simulink model "Simscape_simulink"  (R2024a)
settings: Solver=VariableStepAuto  StartTime=0.0  StopTime=10.0  MaxStep=0.001  RelTol=1e-3
libraries: fl_lib x15, nesl_utility x6, sdl_lib x1
settings Model: Creator=buttrakd  LastModifiedBy=buttrakd

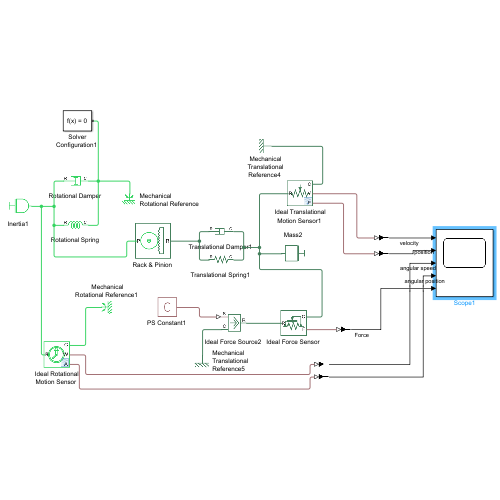
[thumbnail: Simulink's stored preview of the top-level diagram]
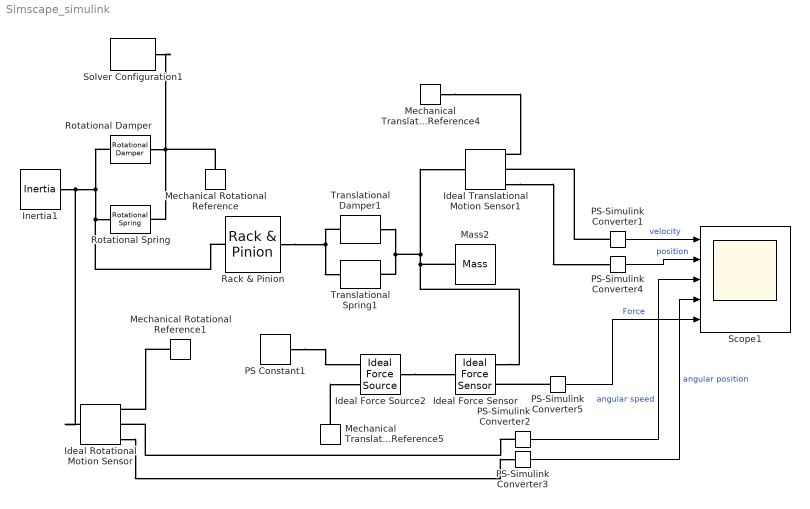
== system Simscape_simulink ==
  "Ideal Force Sensor " : fl_lib/Mechanical/Mechanical Sensors/Ideal Force Sensor
  "Ideal Force Source2 " : fl_lib/Mechanical/Mechanical Sources/Ideal Force Source
  "Ideal Rotational Motion Sensor " : fl_lib/Mechanical/Mechanical Sensors/Ideal Rotational Motion Sensor  reference=foundation.enum.MeasurementReference.difference  acceleration_port=false  velocity_port=true  position_port=true  wrap_angle=false  offset=0 rad
      settings: SimscapeInstrumentationLogging=on
  "Ideal Translational Motion Sensor1 " : fl_lib/Mechanical/Mechanical Sensors/Ideal Translational Motion Sensor  reference=foundation.enum.MeasurementReference.difference  acceleration_port=false  velocity_port=true  position_port=true  offset=0 m
      settings: SimscapeInstrumentationLogging=on
  "Inertia1 " : fl_lib/Mechanical/Rotational Elements/Inertia  inertia=1 kg*m^2  num_ports=foundation.enum.numPorts2.one  w_specify=off  w_priority=High  w=0 rad/s  w_nominal_specify=off  w_nominal_value=1  w_nominal_unit=rad/s  t_specify=off  t_priority=None  t=0 N*m  t_nominal_specify=off  t_nominal_value=1  t_nominal_unit=N*m
  "Mass2 " : fl_lib/Mechanical/Translational Elements/Mass  mass=0.5 kg  num_ports=foundation.enum.numPorts2.one  v_specify=off  v_priority=High  v=0 m/s  v_nominal_specify=off  v_nominal_value=1  v_nominal_unit=m/s  f_specify=off  f_priority=None  f=0 N  f_nominal_specify=off  f_nominal_value=1  f_nominal_unit=N
  "Mechanical Rotational Reference " : fl_lib/Mechanical/Rotational Elements/Mechanical Rotational Reference
  "Mechanical Rotational Reference1 " : fl_lib/Mechanical/Rotational Elements/Mechanical Rotational Reference
  "Mechanical Translational Reference4 " : fl_lib/Mechanical/Translational Elements/Mechanical Translational Reference
  "Mechanical Translational Reference5 " : fl_lib/Mechanical/Translational Elements/Mechanical Translational Reference
  "PS Constant1 " : fl_lib/Physical Signals/Sources/PS Constant  constant=1 N
  PS-Simulink Converter{1..5} (5 alike) : nesl_utility/PS-Simulink Converter  PhysicalDomain=network_engine_domain  SubClassName=ps_output  LeftPortType=input  RightPortType=output  PseudoPeriodic=off  Frequencies=[]  VectorFormat=inherit  Unit=inherit  AffineConversion=off
  "Rack & Pinion " : sdl_lib/Gears/Rotational- Translational/Rack & Pinion  param=sdl.enum.rackPinionParameters.radius  radius=0.4 m  n_teeth=20  x_tooth=5 mm  rack_direction_sign=sdl.enum.pinionDirection.positive  friction_model=sdl.enum.gear_friction.none  efficiency=0.8  temperature_TLU=[280, 300, 320] K  efficiency_TLU=[.95, .9, .85]  pwr_thr=0.001 W  mu_visc_P=0 N*m*s/rad  mu_visc_R=0 N*s/m  thermal_mass=50 J/K  temperature_specify=off  temperature_priority=High  temperature=300 K  temperature_nominal_specify=off  temperature_nominal_value=1  temperature_nominal_unit=K
      settings: InternalSimscapePortConfiguration="{\"Bottom\":[],\"Left\":[{\"id\":\"P\",\"label\":\"P\",\"type\":\"foundation.mechanical.rotational.rotational\"}],\"Right\":[{\"id\":\"R\",\"label\":\"R\",\"type\":\"foundation.mechanical.translational.translational\"}],\"Top\":[]}"
  "Rotational Damper " : fl_lib/Mechanical/Rotational Elements/Rotational Damper  D=0.25 N*m*s/rad  w_specify=off  w_priority=None  w=0 rad/s  w_nominal_specify=off  w_nominal_value=1  w_nominal_unit=rad/s  t_specify=off  t_priority=None  t=0 N*m  t_nominal_specify=off  t_nominal_value=1  t_nominal_unit=N*m
  "Rotational Spring " : fl_lib/Mechanical/Rotational Elements/Rotational Spring  spr_rate=0.5 N*m/rad  w_specify=off  w_priority=None  w=0 rad/s  w_nominal_specify=off  w_nominal_value=1  w_nominal_unit=rad/s  t_specify=off  t_priority=None  t=0 N*m  t_nominal_specify=off  t_nominal_value=1  t_nominal_unit=N*m  phi_specify=off  phi_priority=High  phi=0 rad  phi_nominal_specify=off  phi_nominal_value=1  phi_nominal_unit=rad
  Scope1 : Scope  NumInputPorts=5
  "Solver Configuration1 " : nesl_utility/Solver Configuration  PhysicalDomain=network_engine_domain  SubClassName=solver  LeftPortType=input  RightPortType=generic  Tones=[]  Harmonics=[]  SimulateNoise=off  Profile=off  UseLocalSampling=off  EnableSwitchedLinearOptims=on  FrequencyDomain=off  UseCCode=off  RelTol=0.001  AbsTol=0.001  MinStep=1e-09  ToWorkspace=off  RevertToSquareIcSolve=off  NumHomotopyIterations=100  PhasorMode=off  PhasorModeNumHarmonics=1  ConsistencySolver=NEWTON_XTOL_AFTER_FTOL  IndexReductionMethod=DerivativeReplacement  DoDC=off  ResidualTolerance=1e-09  ConsistencyTolSource=GLOBAL  ConsistencyAbsTol=0.001  ConsistencyRelTol=0.001  ConsistencyTolFactor=0.001  UseLocalSolver=off  LocalSolverChoice=NE_BACKWARD_EULER_ADVANCER  ResolveIndetEquations=on  FunctionEvalNumThread=1  LocalSolverSampleTime=0.001  DoFixedCost=off  MaxNonlinIter=3  MaxModeIter=2  ComputeImpulses=off  ImpulseIterations=2  LinearAlgebra=auto  LinearAlgebraNumThread=0  EquationFormulation=NE_TIME_EF  DelaysMemoryBudget=1024  AutomaticFiltering=on  FilteringTimeConstant=0.001  PartitionStorageMethod=AS_NEEDED  PartitionMemoryBudget=1024  PartitionMethod=ROBUST  MultibodyUseLocalSolver=off  MultibodyLocalSolverChoice=ODE1  MultibodyLocalSolverSampleTime=0.001
  "Translational Damper1 " : fl_lib/Mechanical/Translational Elements/Translational Damper  D=0.25 N*s/m  v_specify=off  v_priority=None  v=0 m/s  v_nominal_specify=off  v_nominal_value=1  v_nominal_unit=m/s  f_specify=off  f_priority=None  f=0 N  f_nominal_specify=off  f_nominal_value=1  f_nominal_unit=N
  "Translational Spring1 " : fl_lib/Mechanical/Translational Elements/Translational Spring  spr_rate=1 N/m  v_specify=off  v_priority=None  v=0 m/s  v_nominal_specify=off  v_nominal_value=1  v_nominal_unit=m/s  f_specify=off  f_priority=None  f=0 N  f_nominal_specify=off  f_nominal_value=1  f_nominal_unit=N  x_specify=off  x_priority=High  x=0 m  x_nominal_specify=off  x_nominal_value=1  x_nominal_unit=m
  wires:
  PS-Simulink Converter1/1 -> Scope1/1  "velocity"
  PS-Simulink Converter2/1 -> Scope1/3  "angular speed"
  PS-Simulink Converter4/1 -> Scope1/2  "position"
  PS-Simulink Converter3/1 -> Scope1/4  "angular position"
  PS-Simulink Converter5/1 -> Scope1/5  "Force"
  connections:
  "Translational Damper1 "/RConn1 -- "Ideal Force Sensor "/RConn1 -- "Mass2 "/LConn1 -- "Ideal Translational Motion Sensor1 "/LConn1 -- "Translational Spring1 "/RConn1
  "Translational Damper1 "/LConn1 -- "Translational Spring1 "/LConn1 -- "Rack & Pinion "/RConn1
  "Mechanical Translational Reference4 "/LConn1 -- "Ideal Translational Motion Sensor1 "/RConn1
  PS-Simulink Converter1/LConn1 -- "Ideal Translational Motion Sensor1 "/RConn2
  "PS Constant1 "/RConn1 -- "Ideal Force Source2 "/RConn1
  "Mechanical Translational Reference5 "/LConn1 -- "Ideal Force Source2 "/RConn2
  "Rotational Damper "/RConn1 -- "Rotational Spring "/RConn1 -- "Solver Configuration1 "/RConn1 -- "Mechanical Rotational Reference "/LConn1
  "Rotational Damper "/LConn1 -- "Ideal Rotational Motion Sensor "/LConn1 -- "Inertia1 "/LConn1 -- "Rack & Pinion "/LConn1 -- "Rotational Spring "/LConn1
  "Mechanical Rotational Reference1 "/LConn1 -- "Ideal Rotational Motion Sensor "/RConn1
  PS-Simulink Converter2/LConn1 -- "Ideal Rotational Motion Sensor "/RConn2
  "Ideal Translational Motion Sensor1 "/RConn3 -- PS-Simulink Converter4/LConn1
  "Ideal Rotational Motion Sensor "/RConn3 -- PS-Simulink Converter3/LConn1
  PS-Simulink Converter5/LConn1 -- "Ideal Force Sensor "/RConn2
  "Ideal Force Source2 "/LConn1 -- "Ideal Force Sensor "/LConn1
